simulink model "flight_model"  (R2019b)
settings: Solver=FixedStepAuto  StartTime=0.0  StopTime=100.0  FixedStep=0.01  RelTol=1e-3
values from neighbouring files (symbols this model uses):
  centerHeigt = 1    [calculator.m]    (also in flight_details.m; landing_dimensions.m; required_speed.m = 0; single_fly.m)
  speed = StartSpeeds(n)    [calculator.m]    (also in flight_details.m = 11.1111111111; landing_dimensions.m; required_speed.m = sqrt(speed^2 + 2*G*rampHeight); single_fly.m = 7)
libraries: simulink x1
settings Model: Creator=Zver  LastModifiedBy=Zver

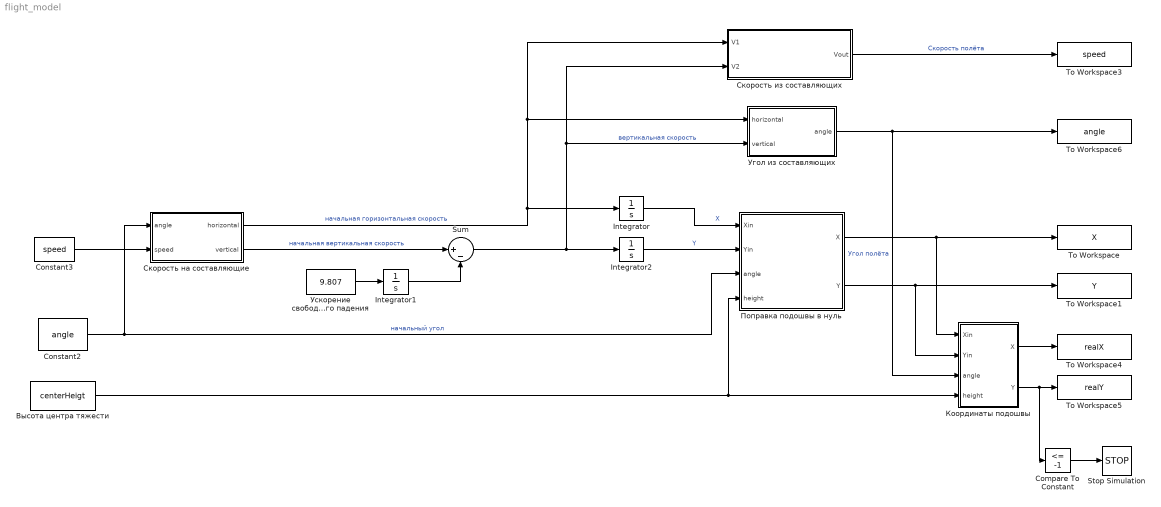
== system flight_model ==
  Compare To Constant : simulink/Logic and Bit Operations/Compare To Constant  relop=<=  const=-1  OutDataTypeStr=boolean
  Constant2 : Constant  Value=angle
  Constant3 : Constant  Value=speed
  Integrator : Integrator
  Integrator1 : Integrator
  Integrator2 : Integrator
  Stop Simulation : Stop
  Sum : Sum  Inputs=|+-
  To Workspace : ToWorkspace  VariableName=X  SaveFormat=Timeseries  SampleTime=-1
  To Workspace1 : ToWorkspace  VariableName=Y  SaveFormat=Timeseries  SampleTime=-1
  To Workspace3 : ToWorkspace  VariableName=speed  SaveFormat=Timeseries  SampleTime=-1
  To Workspace4 : ToWorkspace  VariableName=realX  SaveFormat=Timeseries  SampleTime=-1
  To Workspace5 : ToWorkspace  VariableName=realY  SaveFormat=Timeseries  SampleTime=-1
  To Workspace6 : ToWorkspace  VariableName=angle  SaveFormat=Timeseries  SampleTime=-1
  "Высота центра тяжести " : Constant  Value=centerHeigt
  Координаты подошвы : Subsystem
  Поправка подошвы в нуль : Subsystem
  Скорость из составляющих : Subsystem
  Скорость на составляющие : Subsystem
  Угол из составляющих : Subsystem
  Ускорение свободного падения : Constant  Value=9.807
  wires:
  Ускорение свободного падения/1 -> Integrator1/1
  Sum/1 -> Скорость из составляющих/2(V2), Угол из составляющих/2(vertical), Integrator2/1  "вертикальная скорость"
  Compare To Constant/1 -> Stop Simulation/1
  "Высота центра тяжести "/1 -> Координаты подошвы/4(height), Поправка подошвы в нуль/4(height)
  Constant2/1 -> Скорость на составляющие/1(angle), Поправка подошвы в нуль/3(angle)  "начальный угол"
  Скорость из составляющих/1(Vout) -> To Workspace3/1  "Скорость полёта"
  Координаты подошвы/2(Y) -> Compare To Constant/1, To Workspace5/1
  Координаты подошвы/1(X) -> To Workspace4/1
  Поправка подошвы в нуль/2(Y) -> To Workspace1/1, Координаты подошвы/2(Yin)
  Поправка подошвы в нуль/1(X) -> Координаты подошвы/1(Xin), To Workspace/1
  Integrator2/1 -> Поправка подошвы в нуль/2(Yin)  "Y"
  Integrator/1 -> Поправка подошвы в нуль/1(Xin)  "X"
  Угол из составляющих/1(angle) -> To Workspace6/1, Координаты подошвы/3(angle)  "Угол полёта"
  Скорость на составляющие/1(horizontal) -> Угол из составляющих/1(horizontal), Скорость из составляющих/1(V1), Integrator/1  "начальная горизонтальная скорость"
  Constant3/1 -> Скорость на составляющие/2(speed)
  Скорость на составляющие/2(vertical) -> Sum/1  "начальная вертикальная скорость"
  Integrator1/1 -> Sum/2

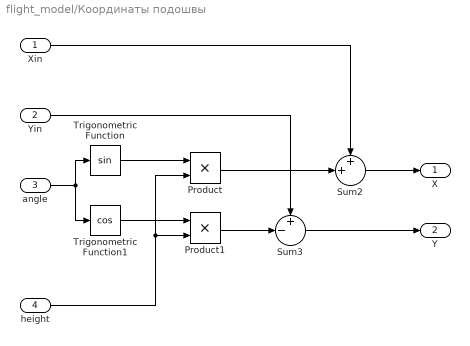
== system flight_model/Координаты подошвы ==
  Xin : Inport
  Yin : Inport  Port=2
  angle : Inport  Port=3
  height : Inport  Port=4
  Product : Product
  Product1 : Product
  Sum2 : Sum  Inputs=++|
  Sum3 : Sum  Inputs=+-|
  Trigonometric Function : Trigonometry
  Trigonometric Function1 : Trigonometry  Operator=cos
  X : Outport
  Y : Outport  Port=2
  wires:
  height/1 -> Product/2, Product1/2
  Trigonometric Function1/1 -> Product1/1
  Product1/1 -> Sum3/2
  Xin/1 -> Sum2/1
  Sum2/1 -> X/1
  Product/1 -> Sum2/2
  Trigonometric Function/1 -> Product/1
  angle/1 -> Trigonometric Function/1, Trigonometric Function1/1
  Yin/1 -> Sum3/1
  Sum3/1 -> Y/1

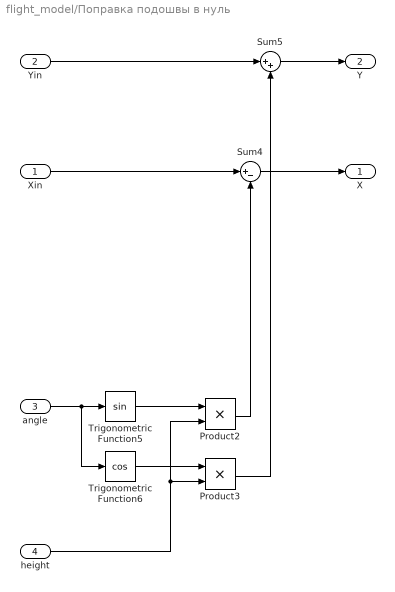
== system flight_model/Поправка подошвы в нуль ==
  Xin : Inport
  Yin : Inport  Port=2
  angle : Inport  Port=3
  height : Inport  Port=4
  Product2 : Product
  Product3 : Product
  Sum4 : Sum  Inputs=|+-
  Sum5 : Sum  Inputs=|++
  Trigonometric Function5 : Trigonometry
  Trigonometric Function6 : Trigonometry  Operator=cos
  X : Outport
  Y : Outport  Port=2
  wires:
  angle/1 -> Trigonometric Function6/1, Trigonometric Function5/1
  Xin/1 -> Sum4/1
  height/1 -> Product3/2, Product2/2
  Trigonometric Function6/1 -> Product3/1
  Product2/1 -> Sum4/2
  Sum5/1 -> Y/1
  Product3/1 -> Sum5/2
  Trigonometric Function5/1 -> Product2/1
  Sum4/1 -> X/1
  Yin/1 -> Sum5/1

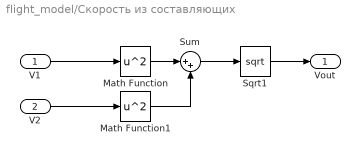
== system flight_model/Скорость из составляющих ==
  V1 : Inport
  V2 : Inport  Port=2
  Math Function : Math  Operator=square  SignedPower=off  SaturateOnIntegerOverflow=on
  Math Function1 : Math  Operator=square  SignedPower=off  SaturateOnIntegerOverflow=on
  Sqrt1 : Sqrt  SaturateOnIntegerOverflow=on
  Sum : Sum  Inputs=|++
  Vout : Outport
  wires:
  Math Function1/1 -> Sum/2
  Math Function/1 -> Sum/1
  Sum/1 -> Sqrt1/1
  Sqrt1/1 -> Vout/1
  V1/1 -> Math Function/1
  V2/1 -> Math Function1/1

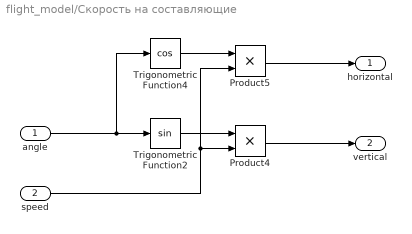
== system flight_model/Скорость на составляющие ==
  angle : Inport
  speed : Inport  Port=2
  Product4 : Product
  Product5 : Product
  Trigonometric Function2 : Trigonometry
  Trigonometric Function4 : Trigonometry  Operator=cos
  horizontal : Outport
  vertical : Outport  Port=2
  wires:
  speed/1 -> Product5/2, Product4/2
  Product5/1 -> horizontal/1
  Trigonometric Function2/1 -> Product4/1
  Trigonometric Function4/1 -> Product5/1
  angle/1 -> Trigonometric Function4/1, Trigonometric Function2/1
  Product4/1 -> vertical/1

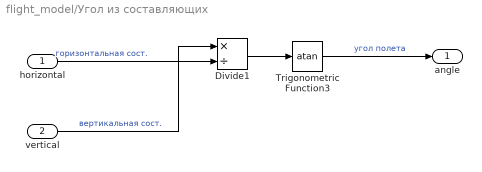
== system flight_model/Угол из составляющих ==
  horizontal : Inport
  vertical : Inport  Port=2
  Divide1 : Product  Inputs=*/
  Trigonometric Function3 : Trigonometry  Operator=atan
  angle : Outport
  wires:
  Trigonometric Function3/1 -> angle/1  "угол полета"
  vertical/1 -> Divide1/1  "вертикальная сост."
  Divide1/1 -> Trigonometric Function3/1
  horizontal/1 -> Divide1/2  "горизонтальная сост."
